simulink model "test_master_task"  (Simulink 3.00)
libraries: mathlib x8, inoutlib x2, logiclib x1

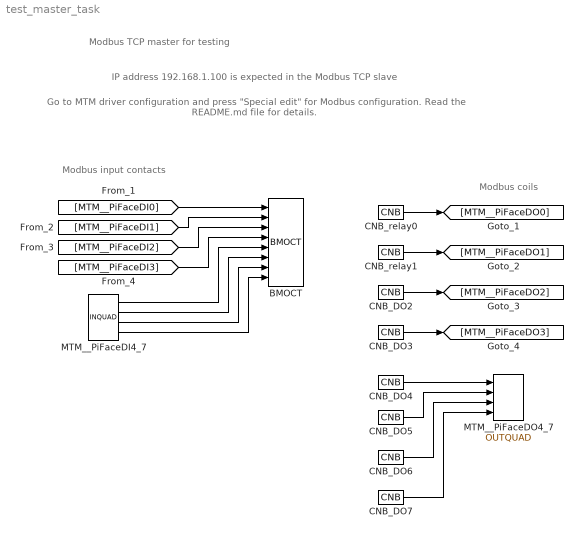
== system test_master_task ==
  note: Modbus TCP master for testing
  note: IP address 192.168.1.100 is expected in the Modbus TCP slave
  note: Go to MTM driver configuration and press "Special edit" for Modbus configuration.
      |
      | Read the README.md file for details.
  note: Modbus input contacts
  note: Modbus coils
  BMOCT : logiclib/BMOCT  shift=0
  CNB_DO{2..7} (6 alike) : mathlib/CNB  YCN=off
  CNB_relay0 : mathlib/CNB  YCN=off
  CNB_relay1 : mathlib/CNB  YCN=off
  MTM__PiFaceDI4_7 : inoutlib/INQUAD
  MTM__PiFaceDO4_7 : inoutlib/OUTQUAD
  wires:
  CNB_DO2/1 -> [MTM__PiFaceDO2]
  CNB_DO3/1 -> [MTM__PiFaceDO3]
  CNB_DO4/1 -> MTM__PiFaceDO4_7/1
  CNB_DO5/1 -> MTM__PiFaceDO4_7/2
  CNB_DO6/1 -> MTM__PiFaceDO4_7/3
  CNB_DO7/1 -> MTM__PiFaceDO4_7/4
  CNB_relay0/1 -> [MTM__PiFaceDO0]
  CNB_relay1/1 -> [MTM__PiFaceDO1]
  [MTM__PiFaceDI0] -> BMOCT/1
  [MTM__PiFaceDI1] -> BMOCT/2
  [MTM__PiFaceDI2] -> BMOCT/3
  [MTM__PiFaceDI3] -> BMOCT/4
  MTM__PiFaceDI4_7/1 -> BMOCT/5
  MTM__PiFaceDI4_7/2 -> BMOCT/6
  MTM__PiFaceDI4_7/3 -> BMOCT/7
  MTM__PiFaceDI4_7/4 -> BMOCT/8
